simulink model "mypid"  (Simulink 7.9)
settings: Solver=ode45  StartTime=0.0  StopTime=100.0  RelTol=1e-3
settings Model: Creator=student  LastModifiedBy=student

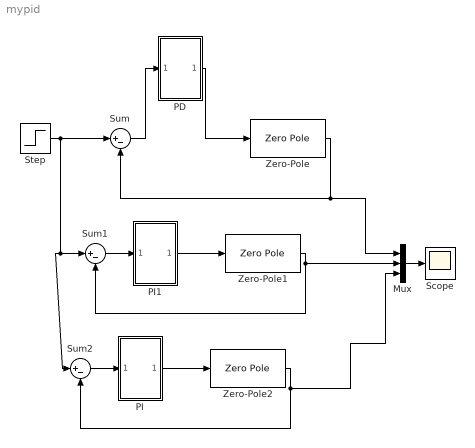
== system mypid ==
  Mux : Mux  Inputs=3
  PD : Subsystem  mask{P=0.5*8, D=0}
  PI : Subsystem  mask{P=0.6*8, I=3.6/2, D=3.6/8}
  PI1 : Subsystem  mask{P=0.45*8, I=3.6/(1.2), D=0}
  Scope : Scope
  Step : Step  SampleTime=0
  Sum : Sum  Inputs=|+-
  Sum1 : Sum  Inputs=|+-
  Sum2 : Sum  Inputs=|+-
  Zero-Pole : ZeroPole  Zeros=[]  Poles=[-1 -1 -1]
  Zero-Pole1 : ZeroPole  Zeros=[]  Poles=[-1 -1 -1]
  Zero-Pole2 : ZeroPole  Zeros=[]  Poles=[-1 -1 -1]
  wires:
  Step/1 -> Sum/1, Sum1/1, Sum2/1
  Sum/1 -> PD/1(In1)
  PD/1(Out1) -> Zero-Pole/1
  Zero-Pole/1 -> Sum/2, Mux/1
  Sum1/1 -> PI1/1(In1)
  PI1/1(Out1) -> Zero-Pole1/1
  Zero-Pole1/1 -> Sum1/2, Mux/2
  Sum2/1 -> PI/1(In1)
  PI/1(Out1) -> Zero-Pole2/1
  Zero-Pole2/1 -> Sum2/2, Mux/3
  Mux/1 -> Scope/1

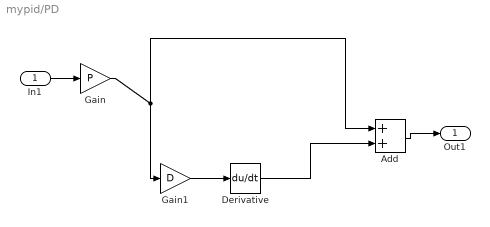
== system mypid/PD ==
  In1 : Inport
  Add : Sum
  Derivative : Derivative
  Gain : Gain  Gain=P
  Gain1 : Gain  Gain=D
  Out1 : Outport
  wires:
  Add/1 -> Out1/1
  Derivative/1 -> Add/2
  Gain1/1 -> Derivative/1
  Gain/1 -> Gain1/1, Add/1
  In1/1 -> Gain/1

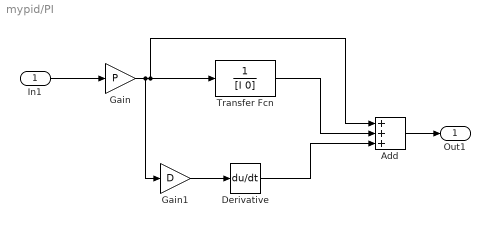
== system mypid/PI ==
  In1 : Inport
  Add : Sum  Inputs=+++
  Derivative : Derivative
  Gain : Gain  Gain=P
  Gain1 : Gain  Gain=D
  Transfer Fcn : TransferFcn  Denominator=[I 0]
  Out1 : Outport
  wires:
  In1/1 -> Gain/1
  Gain/1 -> Gain1/1, Transfer Fcn/1, Add/1
  Gain1/1 -> Derivative/1
  Transfer Fcn/1 -> Add/2
  Derivative/1 -> Add/3
  Add/1 -> Out1/1

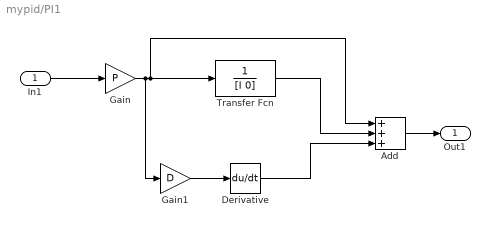
== system mypid/PI1 ==
  In1 : Inport
  Add : Sum  Inputs=+++
  Derivative : Derivative
  Gain : Gain  Gain=P
  Gain1 : Gain  Gain=D
  Transfer Fcn : TransferFcn  Denominator=[I 0]
  Out1 : Outport
  wires:
  In1/1 -> Gain/1
  Gain/1 -> Gain1/1, Transfer Fcn/1, Add/1
  Gain1/1 -> Derivative/1
  Transfer Fcn/1 -> Add/2
  Derivative/1 -> Add/3
  Add/1 -> Out1/1
